simulink model "simulation_lqr_tmp"  (R2021b)
settings: Solver=FixedStepAuto  StartTime=0.0  StopTime=T+10  FixedStep=h  RelTol=1e-3  EnableMultiTasking=on
undefined symbols (not defined in the file or in its folder): constgain, disc, discrete_eq, h, Humusoft, K, MF634, x0
libraries: sldrtlib x2
settings Model: Creator=rbabuska  LastModifiedBy=wterhaar
settings SolverCC: AlgebraicLoopSolver=TrustRegion  AutoInsertRateTranBlk=on
settings DataIOCC: LimitDataPoints=on  SaveFormat=Array  SignalLoggingSaveFormat=ModelDataLogs  SaveOutput=off  SaveTime=off  ReturnWorkspaceOutputs=off
settings OptimizationCC: DefaultParameterBehavior=Inlined  InlineInvariantSignals=on  EnhancedBackFolding=on  PassReuseOutputArgsAs=Individual arguments  ExpressionDepthLimit=2147483647  StateBitsets=on  DataBitsets=on  ZeroExternalMemoryAtStartup=off  ZeroInternalMemoryAtStartup=off  NoFixptDivByZeroProtection=on  LifeSpan=1  OptimizeBlockOrder=speed  DifferentSizesBufferReuse=on  EfficientTunableParamExpr=on
settings DebuggingCC: UnderspecifiedInitializationDetection=Classic  MergeDetectMultiDrivingBlocksExec=none  ParameterTunabilityLossMsg=error  FcnCallInpInsideContextMsg=warning  StateNameClashWarn=warning  SFUnexpectedBacktrackingDiag=warning  SFNoUnconditionalDefaultTransitionDiag=warning  SFExecutionAtInitializationDiag=none  SFMachineParentedDataDiag=warning  ArithmeticOperatorsInVariantConditions=warning
settings HardwareCC: ProdBitPerPointer=32  ProdBitPerSizeT=32  ProdBitPerPtrDiffT=32  ProdLargestAtomicFloat=None  ProdIntDivRoundTo=Floor  ProdWordSize=32  ProdHWDeviceType=Generic->Custom
settings ModelReferenceCC: PropagateSignalLabelsOutOfModel=off
settings SFSimCC: SimUseLocalCustomCode=off  MATLABDynamicMemAlloc=off  CustomCodeUndefinedFunction=UseInterfaceOnly
settings RTWCC: Description=Embedded Coder  SystemTargetFile=ert.tlc  TLCOptions=-p0  GenCodeOnly=on  TemplateMakefile=ert_default_tmf  GenerateReport=on  RTWVerbose=off  RTWUseLocalCustomCode=off  IncludeHyperlinkInReport=on  LaunchReport=on
settings CodeAppCC: ForceParamTrailComments=on  IgnoreCustomStorageClasses=off  OperatorAnnotations=on  SimulinkDataObjDesc=on  SFDataObjDesc=on  CustomSymbolStrGlobalVar=rt$N$M  CustomSymbolStrType=$N$M  CustomSymbolStrFcn=$N$M$F  CustomSymbolStrMacro=$N$M  InsertBlockDesc=on
settings ERTTargetCC: CodeReplacementLibrary=ISO_C  GenerateSampleERTMain=on  IncludeMdlTerminateFcn=off  SuppressErrorStatus=on  SupportAbsoluteTime=off  PurelyIntegerCode=on  SupportNonFinite=off  SupportComplex=off  InlinedParameterPlacement=NonHierarchical  RootIOFormat=Structure reference  ERTCustomFileTemplate=example_file_process.tlc
settings ConfigComp: CovMetricSettings=dw  CovSaveCumulativeToWorkspaceVar=on  CovSaveSingleToWorkspaceVar=on  CovExternalEMLEnable=off  CovSFcnEnable=off

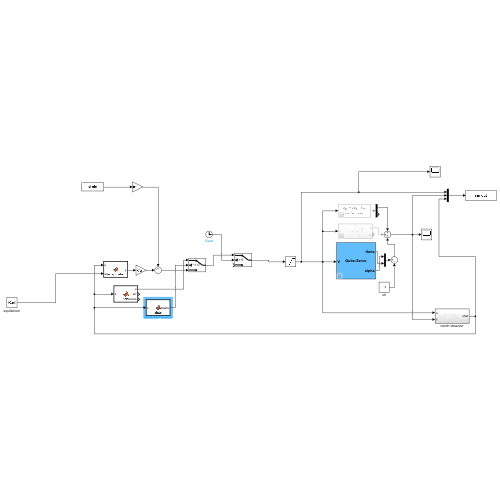
[thumbnail: Simulink's stored preview of the top-level diagram]
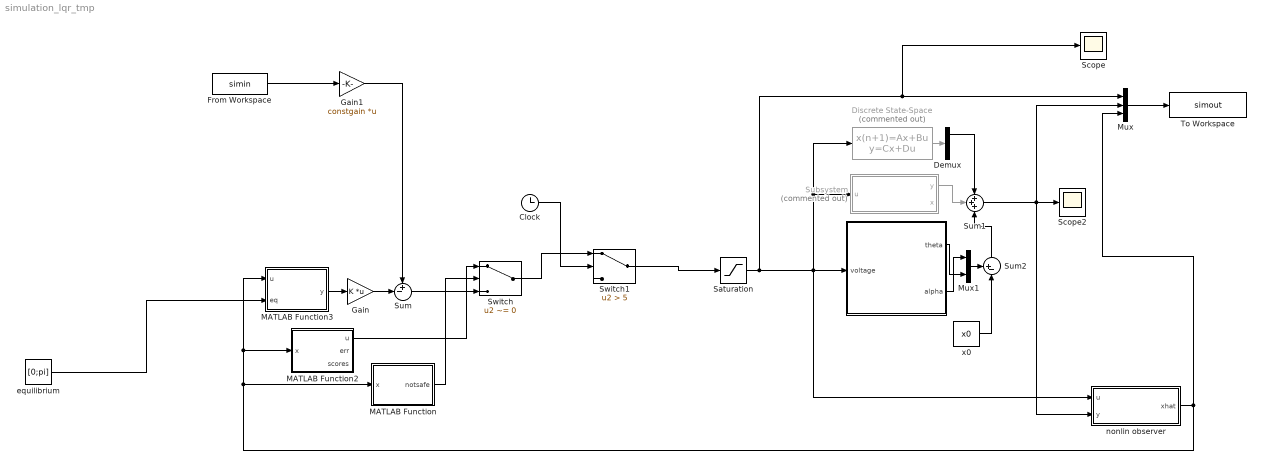
== system simulation_lqr_tmp ==
  " " : Subsystem  LoadFcn=hwinit  InitFcn=hwinit  mask{h=h}
      mask prompts: h "Sampling period [s]"
      mask Display:
      | disp('Qube-Servo')
      | port_label('output',1,'theta')
      | port_label('output',2,'alpha')
      | port_label('input',1,'V')
  Clock : Clock
  Demux : Demux  Outputs=[2;4]
  Discrete State-Space : DiscreteStateSpace  Commented=on  A=discrete_eq.A  B=discrete_eq.B  C=[discrete_eq.C;eye(4)]  D=[discrete_eq.D;zeros(4,1)]  InitialCondition=[0;0;0;0]  SampleTime=h
  From Workspace : FromWorkspace  VariableName=simin  SampleTime=h  OutputAfterFinalValue=Holding final value
  Gain : Gain  Gain=K  Multiplication=Matrix(K*u)
  Gain1 : Gain  Gain=constgain  Multiplication=Matrix(K*u)
  MATLAB Function : MATLAB Function  TreatAsAtomicUnit=on
  MATLAB Function2 : MATLAB Function  TreatAsAtomicUnit=on
  MATLAB Function3 : MATLAB Function  TreatAsAtomicUnit=on
  Mux : Mux  Inputs=3
  Mux1 : Mux  Inputs=2
  Saturation : Saturate  UpperLimit=1  LowerLimit=-1
  Scope : Scope
  Scope2 : Scope
  Subsystem : Subsystem  Commented=on
  Sum : Sum  Inputs=+-|
  Sum1 : Sum  Inputs=+++
  Sum2 : Sum  Inputs=+-|
  Switch : Switch  Criteria=u2 ~= 0
  Switch1 : Switch  Criteria=u2 > Threshold  Threshold=5
  To Workspace : ToWorkspace  VariableName=simout  SaveFormat=Timeseries  SampleTime=-1
  equilibrium : Constant  Value=[0;pi]
  nonlin observer : Subsystem
  x0 : Constant  Value=x0
  wires:
  Mux/1 -> To Workspace/1
  nonlin observer/1(xhat) -> Mux/3, MATLAB Function/1(x), MATLAB Function3/1(u), MATLAB Function2/1(x)
  Discrete State-Space/1 -> Demux/1
  Sum1/1 -> nonlin observer/2(y), Scope2/1, Mux/2
  Saturation/1 -> Discrete State-Space/1, Subsystem/1(u), " "/1(voltage), nonlin observer/1(u), Scope/1, Mux/1
  " "/2(alpha) -> Mux1/1
  " "/1(theta) -> Mux1/2
  Subsystem/1(y) -> Sum1/2
  Demux/1 -> Sum1/1
  From Workspace/1 -> Gain1/1
  Gain/1 -> Sum/2
  Gain1/1 -> Sum/1
  x0/1 -> Sum2/2
  MATLAB Function3/1(y) -> Gain/1
  Mux1/1 -> Sum2/1
  Sum2/1 -> Sum1/3
  MATLAB Function/1(notsafe) -> Switch/2
  equilibrium/1 -> MATLAB Function3/2(eq)
  MATLAB Function2/1(u) -> Switch/1
  Sum/1 -> Switch/3
  Switch/1 -> Switch1/1
  Clock/1 -> Switch1/2
  Switch1/1 -> Saturation/1

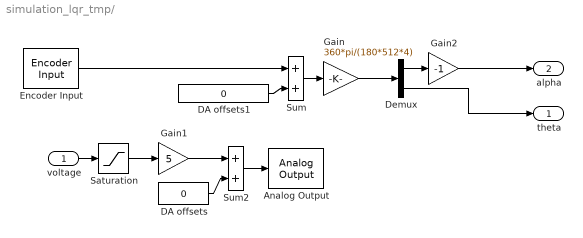
== system simulation_lqr_tmp/  ==
  voltage : Inport
  Analog Output : sldrtlib/Analog Output  SampleTime=h  MaxMissedTicks=100  ShowMissedTicks=off  YieldWhenWaiting=off  DrvName=Humusoft/MF634  DrvAddress=4294967295  DrvOptions=0  Channels=[1]  RangeMode=2  VoltRange=1  InitialValue=0  FinalValue=0
      settings: AttributesFormatString=Humusoft\nMF634 [auto]
  DA offsets : Constant  Value=0
  DA offsets1 : Constant  Value=0  SampleTime=h
  Demux : Demux  Outputs=2
  Encoder Input : sldrtlib/Encoder Input  SampleTime=h  MaxMissedTicks=100  ShowMissedTicks=off  YieldWhenWaiting=off  DrvName=Humusoft/MF634  DrvAddress=4294967295  DrvOptions=0  Channels=[1,2]  QuadMode=3  IndexPulse=1  InputFilter=Inf  DataType=1
      settings: AttributesFormatString=Humusoft\nMF634 [auto]
  Gain : Gain  Gain=360*pi/(180*512*4)  SaturateOnIntegerOverflow=on  OutDataTypeStr=Inherit: Same as input  ParamDataTypeStr=Inherit: Same as input
  Gain1 : Gain  Gain=5  SaturateOnIntegerOverflow=on  OutDataTypeStr=Inherit: Same as input  ParamDataTypeStr=Inherit: Same as input
  Gain2 : Gain  Gain=-1  SaturateOnIntegerOverflow=on  OutDataTypeStr=Inherit: Same as input  ParamDataTypeStr=Inherit: Same as input
  Saturation : Saturate  UpperLimit=1  LowerLimit=-1
  Sum : Sum  InputSameDT=on  SaturateOnIntegerOverflow=on  OutDataTypeStr=Inherit: Same as first input
  Sum2 : Sum  InputSameDT=on  SaturateOnIntegerOverflow=on  OutDataTypeStr=Inherit: Same as first input
  theta : Outport  Tag=Cable length
  alpha : Outport  Tag=Cable length  Port=2
  wires:
  Sum/1 -> Gain/1
  DA offsets1/1 -> Sum/2
  Gain1/1 -> Sum2/1
  Sum2/1 -> Analog Output/1
  DA offsets/1 -> Sum2/2
  voltage/1 -> Saturation/1
  Encoder Input/1 -> Sum/1
  Saturation/1 -> Gain1/1
  Demux/1 -> Gain2/1
  Gain/1 -> Demux/1
  Gain2/1 -> alpha/1
  Demux/2 -> theta/1

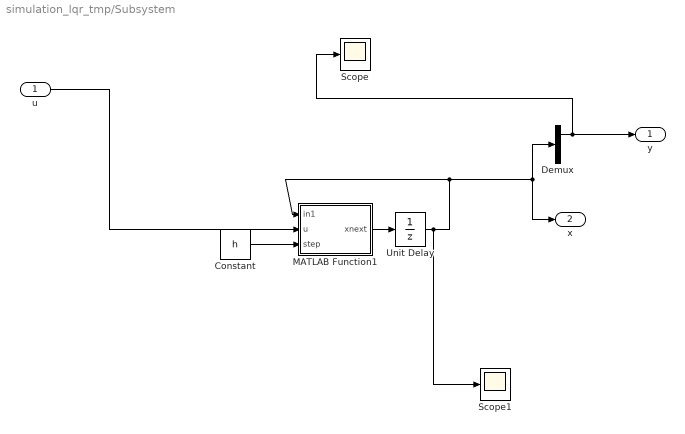
== system simulation_lqr_tmp/Subsystem ==
  u : Inport
  Constant : Constant  Value=h
  Demux : Demux  Outputs=[2,2]
  MATLAB Function1 : MATLAB Function  TreatAsAtomicUnit=on
  Scope : Scope
  Scope1 : Scope
  Unit Delay : UnitDelay  InitialCondition=[x0;0;0]  SampleTime=h  HasFrameUpgradeWarning=on
  y : Outport  PortDimensions=2
  x : Outport  Port=2  PortDimensions=4
  wires:
  u/1 -> MATLAB Function1/2(u)
  Unit Delay/1 -> Scope1/1, MATLAB Function1/1(in1), Demux/1, x/1
  MATLAB Function1/1(xnext) -> Unit Delay/1
  Constant/1 -> MATLAB Function1/3(step)
  Demux/1 -> Scope/1, y/1

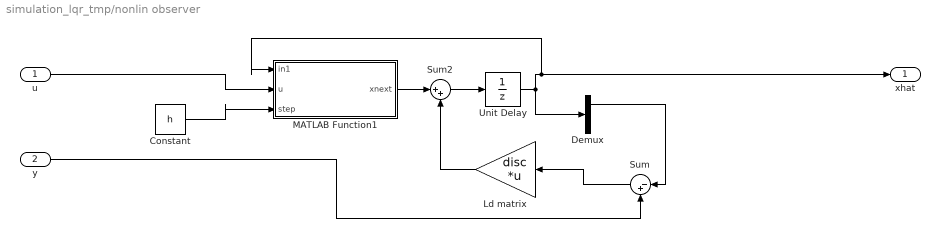
== system simulation_lqr_tmp/nonlin observer ==
  u : Inport  PortDimensions=1
  y : Inport  Port=2  PortDimensions=2
  Constant : Constant  Value=h
  Demux : Demux  Outputs=[2,2]
  Ld matrix : Gain  Gain=disc  Multiplication=Matrix(K*u)
  MATLAB Function1 : MATLAB Function  TreatAsAtomicUnit=on
  Sum : Sum  Inputs=|-+
  Sum2 : Sum  Inputs=|++
  Unit Delay : UnitDelay  InitialCondition=[x0;0;0]  SampleTime=h  HasFrameUpgradeWarning=on
  xhat : Outport  PortDimensions=4
  wires:
  u/1 -> MATLAB Function1/2(u)
  y/1 -> Sum/2
  Sum/1 -> Ld matrix/1
  Constant/1 -> MATLAB Function1/3(step)
  Demux/1 -> Sum/1
  Unit Delay/1 -> MATLAB Function1/1(in1), xhat/1, Demux/1
  MATLAB Function1/1(xnext) -> Sum2/1
  Sum2/1 -> Unit Delay/1
  Ld matrix/1 -> Sum2/2

== matlab function simulation_lqr_tmp/MATLAB Function ==
  data: x input; notsafe output
function notsafe = state(x)
time=0;
futureangle=x(2)+time*x(4);

neartop=abs(wrapToPi(futureangle-pi))<27/180*pi;%10deg from top
% slowtheta=abs(u(4))<30/180*pi;%10deg/sec
notsafe=double(~neartop);

== matlab function simulation_lqr_tmp/MATLAB Function2 ==
  data: x input; u output; err output; scores output
function [u, err, scores] = fcn(x)

%generated in EOM_script.m
stepx=@(in1,u,step)[in1(1,:)+in1(3,:).*step;in1(2,:)+step.*in1(4,:);in1(3,:)-(step.*(in1(1,:).*-2.411134186239272e+40-in1(3,:).*3.153193693480702e+39+u.*1.11324565521834e+42+in1(4,:).^2.*sin(in1(2,:)).*7.93670026513626e+38+cos(in1(2,:)).*sin(in1(2,:)).*9.495003609876428e+40+in1(4,:).*cos(in1(2,:)).*7.869026636066092e+37))./(cos(in1(2,:)).^2.*8.227067348007099e+38-1.634792425014755e+39);in1(4,:)+(step.*(in1(4,:).*1.723890861921848e+57+sin(in1(2,:)).*2.08009843072076e+60-in1(1,:).*cos(in1(2,:)).*2.658230083953888e+59-in1(3,:).*cos(in1(2,:)).*3.476336731643141e+58+u.*cos(in1(2,:)).*1.227332393369617e+61+in1(4,:).^2.*cos(in1(2,:)).*sin(in1(2,:)).*8.750062743300325e+57))./(cos(in1(2,:)).^2.*8.750062743300325e+57-1.738716323334376e+58)];
energy=@(in1)cos(in1(2,:)).*(-1.447956e-2)+(in1(3,:).*(1.7e+1./2.0e+2)+in1(4,:).*cos(in1(2,:)).*6.15e-2).^2.*(3.0./2.5e+2)+in1(4,:).^2.*sin(in1(2,:)).^2.*4.5387e-5+in1(4,:).^2.*1.5129e-5+1.447956e-2;
massoffset=@(in1)in1(1,:).*2.125021070206347e-3+sin(in1(2,:)).*1.2546e-4;

err=massoffset(x);

inputs=-0.5:0.1:0.5;

% inputs=max(min(inputs,0.5),-0.5);
uoff=-800*err;
inputs=inputs+uoff;

etarget=energy([0;pi;0;0])*0.92;

steptime=0.01;
scorebest=1000000;
ubest=0;

scores=zeros(size(inputs));
i=1;
for u=inputs
    xnew=stepx(x,u,steptime);
    score=abs(energy(xnew)-etarget);
%     score=-energy(xnew);
    if score<scorebest
        ubest=u;
        scorebest=score;
    end
    scores(i)=score;
    i=i+1;
end

uenergy=ubest;

u=uenergy;

== matlab function simulation_lqr_tmp/MATLAB Function3 ==
  data: u input; y output; eq input
function y = wraptheta(u,eq)
y=u-[eq;0;0];
y(2)=wrapToPi(y(2));

== matlab function simulation_lqr_tmp/Subsystem/MATLAB Function1 ==
  data: in1 input; u input; xnext output; step input
function xnext = generated_nonlineuler(in1,u,step)
%GENERATED_NONLINEULER
%    XNEXT = GENERATED_NONLINEULER(IN1,U,STEP)

%    This function was generated by the Symbolic Math Toolbox version 9.0.
%    21-Oct-2022 12:39:30

alpha = in1(1,:);
alpha_dot = in1(3,:);
theta = in1(2,:);
theta_dot = in1(4,:);
t2 = cos(theta);
t3 = sin(theta);
t4 = theta_dot.^2;
t5 = t2.^2;
t6 = t5.*1.874218020926506e+20;
t7 = t6-3.724240113555168e+20;
t8 = 1.0./t7;
et1 = alpha.*-2.411134186239272e+40-alpha_dot.*3.153193693480702e+39+u.*1.11324565521834e+42+t2.*t3.*9.495003609876428e+40;
et2 = t3.*t4.*7.93670026513626e+38+t2.*theta_dot.*7.869026636066092e+37;
et3 = t3.*2.08009843072076e+60+theta_dot.*1.723890861921848e+57-alpha.*t2.*2.658230083953888e+59;
et4 = alpha_dot.*t2.*-3.476336731643141e+58+t2.*u.*1.227332393369617e+61+t2.*t3.*t4.*8.750062743300325e+57;
xnext = [alpha+alpha_dot.*step;theta+step.*theta_dot;alpha_dot-(step.*t8.*(et1+et2))./4.389599959101935e+18;theta_dot+(step.*t8.*(et3+et4))./4.668647214786035e+37];

== matlab function simulation_lqr_tmp/nonlin observer/MATLAB Function1 ==
  data: in1 input; u input; xnext output; step input
function xnext = generated_nonlineuler(in1,u,step)
%GENERATED_NONLINEULER
%    XNEXT = GENERATED_NONLINEULER(IN1,U,STEP)

%    This function was generated by the Symbolic Math Toolbox version 9.0.
%    21-Oct-2022 12:39:30

alpha = in1(1,:);
alpha_dot = in1(3,:);
theta = in1(2,:);
theta_dot = in1(4,:);
t2 = cos(theta);
t3 = sin(theta);
t4 = theta_dot.^2;
t5 = t2.^2;
t6 = t5.*1.874218020926506e+20;
t7 = t6-3.724240113555168e+20;
t8 = 1.0./t7;
et1 = alpha.*-2.411134186239272e+40-alpha_dot.*3.153193693480702e+39+u.*1.11324565521834e+42+t2.*t3.*9.495003609876428e+40;
et2 = t3.*t4.*7.93670026513626e+38+t2.*theta_dot.*7.869026636066092e+37;
et3 = t3.*2.08009843072076e+60+theta_dot.*1.723890861921848e+57-alpha.*t2.*2.658230083953888e+59;
et4 = alpha_dot.*t2.*-3.476336731643141e+58+t2.*u.*1.227332393369617e+61+t2.*t3.*t4.*8.750062743300325e+57;
xnext = [alpha+alpha_dot.*step;theta+step.*theta_dot;alpha_dot-(step.*t8.*(et1+et2))./4.389599959101935e+18;theta_dot+(step.*t8.*(et3+et4))./4.668647214786035e+37];
